simulink model "motor_model_simulink"  (R2022b)
settings: Solver=VariableStepAuto  StartTime=0.0  StopTime=10  RelTol=1e-3
libraries: cstblocks x3
settings Model: Creator=you29  LastModifiedBy=you29

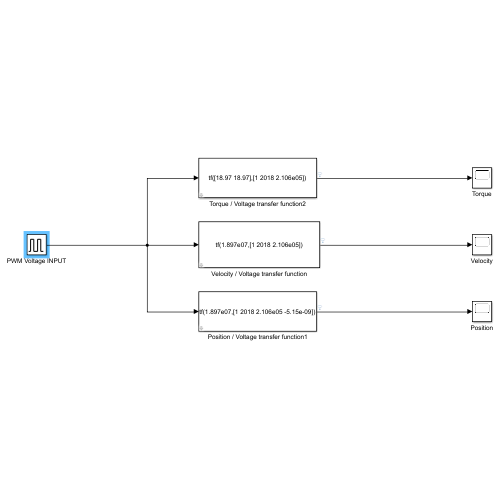
[thumbnail: Simulink's stored preview of the top-level diagram]
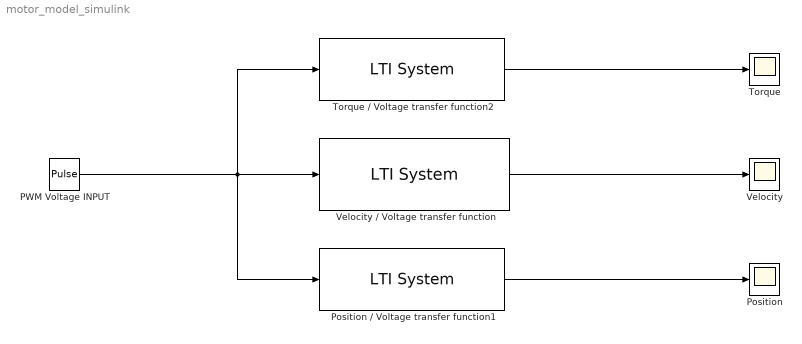
== system motor_model_simulink ==
  PWM Voltage INPUT : DiscretePulseGenerator  PulseType=Time based  Amplitude=12  Period=1  PulseWidth=80
  Position : Scope
  Position / Voltage transfer function1 : cstblocks/LTI System  sys=tf(1.897e07,[1 2018 2.106e05 -5.15e-09])  IC=[]
  Torque : Scope
  Torque / Voltage transfer function2 : cstblocks/LTI System  sys=tf([18.97 18.97],[1 2018 2.106e05])  IC=[]
  Velocity : Scope
  Velocity / Voltage transfer function : cstblocks/LTI System  sys=tf(1.897e07,[1 2018 2.106e05])  IC=[]
  wires:
  PWM Voltage INPUT/1 -> Torque / Voltage transfer function2/1, Position / Voltage transfer function1/1, Velocity / Voltage transfer function/1
  Velocity / Voltage transfer function/1 -> Velocity/1
  Position / Voltage transfer function1/1 -> Position/1
  Torque / Voltage transfer function2/1 -> Torque/1
